simulink model "pid_control"  (R2022a)
settings: Solver=VariableStepAuto  StartTime=0.0  StopTime=10.0  RelTol=1e-3
settings Model: Creator=root  LastModifiedBy=root

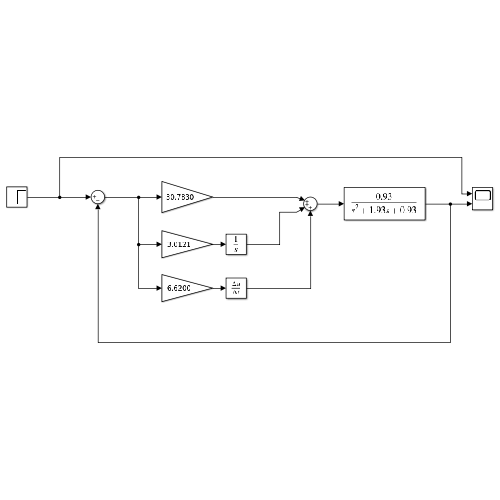
[thumbnail: Simulink's stored preview of the top-level diagram]
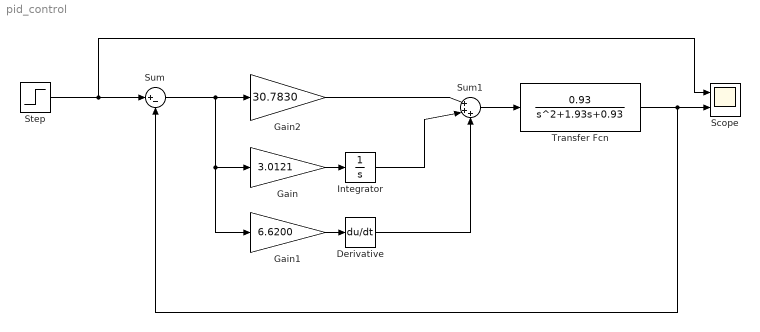
== system pid_control ==
  Derivative : Derivative
  Gain : Gain  Gain=3.0121
  Gain1 : Gain  Gain=6.6200
  Gain2 : Gain  Gain=30.7830
  Integrator : Integrator
  Scope : Scope  NumInputPorts=2
  Step : Step  SampleTime=0
  Sum : Sum  Inputs=|+-
  Sum1 : Sum  Inputs=|+++
  Transfer Fcn : TransferFcn  Numerator=[0.93]  Denominator=[1 1.93 0.93]
  wires:
  Gain1/1 -> Derivative/1
  Gain/1 -> Integrator/1
  Sum1/1 -> Transfer Fcn/1
  Gain2/1 -> Sum1/1
  Integrator/1 -> Sum1/2
  Derivative/1 -> Sum1/3
  Transfer Fcn/1 -> Scope/2, Sum/2
  Step/1 -> Scope/1, Sum/1
  Sum/1 -> Gain1/1, Gain/1, Gain2/1
